simulink model "TJ1000_In_Flight_Start"  (R2019a)
settings: Solver=FixedStepAuto  StartTime=0.0  StopTime=100  FixedStep=0.2  RelTol=1e-3
settings Model: Creator=anton  LastModifiedBy=anton

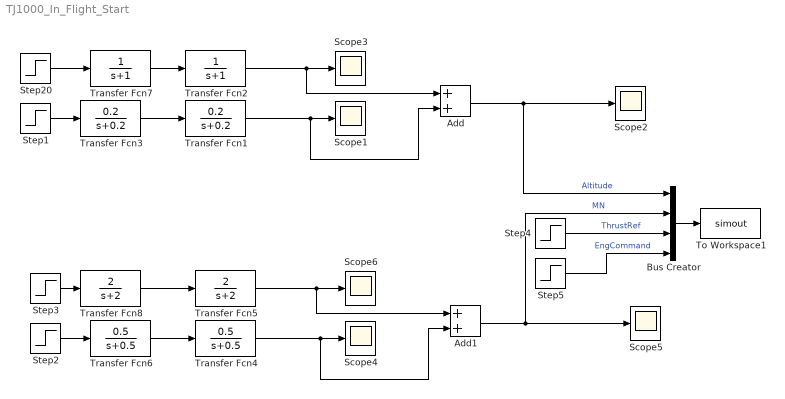
== system TJ1000_In_Flight_Start ==
  Add : Sum
  Add1 : Sum
  Bus Creator : BusCreator  Inputs=4
  Scope{1..6} (6 alike) : Scope
  Step1 : Step  Time=10  After=-200  SampleTime=0
  Step2 : Step  Time=4  After=-0.4  SampleTime=0
  Step20 : Step  After=400  SampleTime=0
  Step3 : Step  After=0.5  SampleTime=0
  Step4 : Step  After=3500  SampleTime=0
  Step5 : Step  Time=0  After=170  SampleTime=0
  To Workspace1 : ToWorkspace  VariableName=simout  SaveFormat=Timeseries  SampleTime=-1
  Transfer Fcn1 : TransferFcn  Numerator=0.2  Denominator=[1 0.2]
  Transfer Fcn2 : TransferFcn  Numerator=1  Denominator=[1 1]
  Transfer Fcn3 : TransferFcn  Numerator=0.2  Denominator=[1 0.2]
  Transfer Fcn4 : TransferFcn  Numerator=0.5  Denominator=[1 0.5]
  Transfer Fcn5 : TransferFcn  Numerator=2  Denominator=[1 2]
  Transfer Fcn6 : TransferFcn  Numerator=0.5  Denominator=[1 0.5]
  Transfer Fcn7 : TransferFcn  Numerator=1  Denominator=[1 1]
  Transfer Fcn8 : TransferFcn  Numerator=2  Denominator=[1 2]
  wires:
  Step20/1 -> Transfer Fcn7/1
  Transfer Fcn2/1 -> Add/1, Scope3/1
  Step1/1 -> Transfer Fcn3/1
  Transfer Fcn1/1 -> Add/2, Scope1/1
  Add/1 -> Bus Creator/1, Scope2/1  "Altitude"
  Transfer Fcn3/1 -> Transfer Fcn1/1
  Transfer Fcn6/1 -> Transfer Fcn4/1
  Add1/1 -> Bus Creator/2, Scope5/1  "MN"
  Transfer Fcn4/1 -> Scope4/1, Add1/2
  Step2/1 -> Transfer Fcn6/1
  Transfer Fcn5/1 -> Scope6/1, Add1/1
  Step3/1 -> Transfer Fcn8/1
  Transfer Fcn7/1 -> Transfer Fcn2/1
  Transfer Fcn8/1 -> Transfer Fcn5/1
  Bus Creator/1 -> To Workspace1/1
  Step4/1 -> Bus Creator/3  "ThrustRef"
  Step5/1 -> Bus Creator/4  "EngCommand"
